simulink model "irep_force_control_m15"  (R2015a)
settings: Solver=ode3  StartTime=0.0  StopTime=inf  FixedStep=dt  RelTol=1e-3
InitFcn:
  | IREP_DEPENDENCY
  | init_omni
  | init_filters
  | init_invivo
  | init_telemanipulation
  | init_parker_xyz
  | init_magnetic_tracker
  | init_loadcell
  | init_scopes
  | init_homing
  | init_force_control
  | init_xpc_invivo_simu
undefined symbols (not defined in the file): ang_vel_scale, B_simu, beta, camera_home_voltage, counter_offset, dt, dt_trakstar, E_Y, encoder_counts, epsilon_robust_inverse, FS_LUT_TAU, FS_LUT_WE, gear_ratio, HomingFineEps, HomingRoughEps, HomingRoughVelocity, I1_primary, I1_secondary, I2_primary, I2_secondary, irep_parameters_left, irep_parameters_right, joystick_filter_coeffs, K_d, K_i, K_naive_inv, K_p, k_right, L1l, L1r, L2l, L2r, L_zeus, left_arm_home_voltage, left_x0_parallelogram, LeftArmHomingDirectionVector, LeftArmHomingIntGain, lin_vel_scale, LOADCELL_BIAS, LOADCELL_GAIN, max_conf_space_speed, N_joystick, N_pots, N_trakstar, OmegaMax, OmegaMin, orientation_epsilon, position_epsilon, pots_filter_coeffs, q_eps_backlash, quadrature_mode, r, right_arm_home_voltage, RightArmHomingDirectionVector, RightArmHomingIntGain, screw_pitch, statics_param, tau_compression_bias, tau_compression_gains, tau_neutral_deadband ... (+16)
libraries: slrtlib x39, simulink x23, xpcobsoletelib x23, xpcconteclib x23, xpcrtudplib x12, xpcmeasurementcomputinglib x6, dspswit3 x2, dspsigops x1
(part 7 of 7)

== matlab function irep_force_control_m15/Trajectory Planner/Right Arm/Low Level/Home Procedure/Fine_Rough_Homing_Switch ==
  data: EnableFineHoming output; error input; dt input; q_des output; ERROR_eps input; HomingVel input; q_cur input; HomedJoint output boolean; PrevHomedJoint input boolean
function [EnableFineHoming,q_des,HomedJoint] = fcn(error, dt,ERROR_eps,HomingVel,q_cur,PrevHomedJoint)
%#eml
%   By Long Wang, 2015/1/20
%   Input:
%       error       -> the current error in potentiometers
%       ERROR_eps   -> the tolenrace defined in potentiometers which will determine if within rough control range 
%       q_cur       -> the previous command
%       PrevHomedJoint  -> if homed detected from the previous time step
%       HomingVel       -> the joint velocity to command if the joint is rough homing mode
HomedJoint = (abs(error)<ERROR_eps);
HomedJoint = (HomedJoint|PrevHomedJoint); 
%   if the joint was detected homed previously, it will be forever seen as homed
%   to avoid noise on pots.
if sum(HomedJoint)==9
    % all joints are in rough homing control range, need to use fine homing
    q_des = q_cur; % stays the previous command
    EnableFineHoming = 1;
else
    %   not all joints are in rough homing control range
    %   the ones which are not, need to give constant velocity command
    %   And the other joints will be waiting untill all the joints are in Fine Homing mode
    EnableFineHoming = 0;
    velocity = (1-HomedJoint).*sign(error).*HomingVel; 
    q_des = q_cur + velocity*dt;
end

== matlab function irep_force_control_m15/Wrench Estimation/Wrench Est Right Arm/compute wrench est ==
  data: Ws output; W_seg1 output; tau_curr input; Psi input; n_t input; n_n input; c_t input; c_n input; L input; r input; statics_param input; probe_offset input
function [Ws,W_seg1] = fcn(tau_curr,Psi,n_t,n_n,c_t,c_n,L,r,statics_param,probe_offset)
%#eml
q = in_vivo_invkin(Psi,r);
[Ws,W_seg1] = ...
    right_arm_wrench_estimation(tau_curr,...
    q,Psi,...
    n_t,n_n,...
    c_t,c_n,...
    L,r,...
    statics_param,...
    probe_offset);

== matlab function irep_force_control_m15/Trajectory Planner/Left Arm/Low Level/Home Procedure/Fine_Rough_Homing_Switch ==
  data: EnableFineHoming output; error input; dt input; q_des output; ERROR_eps input; HomingVel input; q_cur input; HomedJoint output boolean; PrevHomedJoint input boolean
function [EnableFineHoming,q_des,HomedJoint] = fcn(error, dt,ERROR_eps,HomingVel,q_cur,PrevHomedJoint)
%#eml
%   By Long Wang, 2015/1/20
%   Input:
%       error       -> the current error in potentiometers
%       ERROR_eps   -> the tolenrace defined in potentiometers which will determine if within rough control range 
%       q_cur       -> the previous command
%       PrevHomedJoint  -> if homed detected from the previous time step
%       HomingVel       -> the joint velocity to command if the joint is rough homing mode
HomedJoint = (abs(error)<ERROR_eps);
HomedJoint = (HomedJoint|PrevHomedJoint); 
%   if the joint was detected homed previously, it will be forever seen as homed
%   to avoid noise on pots.
if sum(HomedJoint)==9
    % all joints are in rough homing control range, need to use fine homing
    q_des = q_cur; % stays the previous command
    EnableFineHoming = 1;
else
    %   not all joints are in rough homing control range
    %   the ones which are not, need to give constant velocity command
    %   And the other joints will be waiting untill all the joints are in Fine Homing mode
    EnableFineHoming = 0;
    velocity = (1-HomedJoint).*sign(error).*HomingVel; 
    q_des = q_cur + velocity*dt;
end

== matlab function irep_force_control_m15/Trajectory Planner/Left Arm/Low Level/Home Procedure/Homing Flags/Homing Completion ==
  data: u input; Homed output; EPS input; dt input; Homed_T output; Homed_T_prev input
function [Homed,Homed_T] = fcn(u,EPS,dt,Homed_T_prev)
%#eml
Homed_T = zeros(9,1);
u = abs(u);
Homed = (u<=EPS);
for i=1:9
    if Homed(i)
        Homed_T(i) = Homed_T_prev(i) + dt; %increment timer
    else
        Homed_T(i) = 0; % reset timer
    end
end

== matlab function irep_force_control_m15/Trajectory Planner/Left Arm/High Level/Task Space/Desired Twist Module/Compute Twist ==
  data: p_des input; R_des input; MSG_Type input; x_des output; p_curr input; R_curr input; Vmax input; Vmin input; position_epsilon input; lin_vel_scale input; OmegaMax input; OmegaMin input; orientation_epsilon input; ang_vel_scale input; theta output
function [x_des,theta] = fcn(p_des,R_des,MSG_Type,p_curr,R_curr,Vmax,Vmin,position_epsilon,lin_vel_scale,OmegaMax,OmegaMin,orientation_epsilon,ang_vel_scale)
%--------------------------------------------------------------------------
% decode the message_type
% MSG_Type def
% bit0 = valid massage or not(enable or not)
% bit1 = time stamping requested or not (if should send back the local time or not)
enable = bitand(uint8(floor(MSG_Type)),1);
% position
% theta_err = 0;
position_error = p_des-p_curr;
M = norm(position_error);
% orientation
R = R_curr'*R_des;
theta = acos((R(1,1)+R(2,2)+R(3,3)-1)/2);
if isnan(theta)
    theta = 0;
%     theta_err = 1;
end
%----------------------------------------------------------------------
if enable == 1
    if M < position_epsilon && theta < orientation_epsilon
        x_des = zeros(6,1);
    else
        n = position_error/M;
        r_non_unit = [R(3,2)-R(2,3);R(1,3)-R(3,1);R(2,1)-R(1,2)];
        if sum(r_non_unit) == 0
            r = zeros(3,1);
        else
            r = r_non_unit/norm(r_non_unit);
        end
        if M > lin_vel_scale*position_epsilon
            LinVelMag = Vmax; % mm/s
        else
            LinVelMag = M*(Vmax-Vmin)/(position_epsilon*(lin_vel_scale-1)) + (lin_vel_scale*Vmin-Vmax)/(lin_vel_scale-1);
        end
        if theta > ang_vel_scale * orientation_epsilon
            AngVelMag = OmegaMax;
        else
            AngVelMag = theta*(OmegaMax-OmegaMin)/(orientation_epsilon*(ang_vel_scale-1))+ (ang_vel_scale*OmegaMin-OmegaMax)/(ang_vel_scale-1);
        end
        x_des = [LinVelMag*n
                 AngVelMag*r];
    end
else
    x_des = zeros(6,1);
end

== matlab function irep_force_control_m15/Trajectory Planner/Right Arm/High Level/Actuation Compensation/q_eps 5th order poly/Embedded MATLAB Function ==
  data: p_des input; p_curr input; tf input; tc input; p output; pdot output; conf input; confn output; t0 input; t0n output; p0n output; p0 input; enable input
function [p,pdot,confn,t0n,p0n] = fifth_order_p(p_des,p_curr,tf,tc,conf,t0,p0,enable)

if enable == 0                  % Configuration space is not used (pdot = 0). 
    p = p_curr;          % However we do want to record the current 
    confn = 0;                  % position in order to be ready as soon 
    t0n = tc;                   % as the enable becomes 1. 
    p0n = p_curr;
    pdot = zeros(9,1);
else
    if (p_des-p0)'*(p_des-p0) > 0
        if conf == 0                % conf = 0 means that the 5th order poly 
            p0n = p0;               % is not configured for the desired trajectory.
            t0n = tc;               % Therefore, the block is initialized.
            confn = 1;
            p = p0;
            pdot = zeros(9,1);
        else
            p0n = p0;
            t0n = t0;
            confn = conf;
            % 5th order polynomial
            a0 = p0;
            a4 = -15*(p_des-p0);
            a3 = -2/3 * a4;
            a5 = -2/5 * a4;
            t = tc-t0;
            tau = t/tf;
            if t < tf
                p = a0 + a3 * tau^3 + a4 * tau^4 + a5 * tau^5;
                pdot = 3*a3*t^2/tf^3 + 4*a4*t^3/tf^4 + 5*a5*t^4/tf^5;
            else
                p = p_des;
                pdot = zeros(9,1);
                p0n = p_des;
            end
        end
    else
        p = p_des;
        pdot = zeros(9,1);
        confn = 0;
        p0n = p0;
        t0n = t0;
    end
end
%------------------------------------------------------------------------

== matlab function irep_force_control_m15/Trajectory Planner/Right Arm/High Level/Actuation Compensation/RR Act Compensation ==
  data: conf_space input; eps output; q_dot input
function eps= RR_Act_Comp(conf_space,q_dot)
%#codegen
% Edited by Rajarshi Roy
% Last Updated: 12/1/2015
% Compensation initialization
eps = zeros(9,1); 
% Compensation correction
flag_direction = 1; % this flag_direction has been abandoned. not being used.
eps([4,5,6,7],1) = RRComputeActuation(flag_direction,conf_space,q_dot);

== matlab function irep_force_control_m15/Dual daVinci MTM/MTML/Embedded MATLAB Function ==
  data: R_vec input; R output
function R = parse_rot(R_vec)
%#eml
R = reshape(R_vec,3,3);

== matlab function irep_force_control_m15/In-Vivo System/Magnetic Tracker 125 Hz/Process sensors ==
  data: BaseX_sr input; psi output; BaseZ_sr input; Seg1_Z_sr input; Seg2_Z_sr input; theta_eps input; error_flag output
function [psi,error_flag] = fcn(BaseX_sr,BaseZ_sr,Seg1_Z_sr,Seg2_Z_sr,theta_eps)
%#eml
[psi,error_flag] = get_psi_measured_2segments(BaseX_sr,BaseZ_sr,Seg1_Z_sr,Seg2_Z_sr,theta_eps);

== matlab function irep_force_control_m15/Dual daVinci MTM/Task Space Command/Right Arm - 5th Order Polynomial and Slerp/Embedded MATLAB Function1 ==
  data: quat output; quat_f input; quat_curr input; tf input; tc input; conf input; confn output; t0 input; t0n output; quat0n output; quat0 input; enable input; RECORD output
function [quat,confn,t0n,quat0n,RECORD] = quat_slerp(quat_f,quat_curr,tf,tc,conf,t0,quat0,enable)
%%  modified version of 5th order poly for Slerp
%   
RECORD = 0;
if enable == 0                  % Configuration space is not used (pdot = 0). 
    quat = quat_curr;
    confn = 0;                  % position in order to be ready as soon 
    t0n = tc;                   % as the enable becomes 1. 
    quat0n = quat_curr;
else
    if (quat0'*quat_f)<1
        if conf == 0                % conf = 0 means that the 5th order poly 
            quat0n = quat0;               % is not configured for the desired trajectory.
            t0n = tc;               % Therefore, the block is initialized.
            confn = 1;
            quat = quat0;
        else
            quat0n = quat0;
            t0n = t0;
            confn = conf;
            % Slerp
            t = tc-t0;
            tau = t/tf;
            if t < tf
                RECORD = 1;
                quat = slerp(quat0,quat_f,tau);
            else
                quat = quat_f;
                quat0n = quat_f;
            end
        end
    else
        quat = quat_f;
        confn = 0;
        quat0n = quat0;
        t0n = t0;
    end
end
%------------------------------------------------------------------------

== matlab function irep_force_control_m15/Trajectory Planner/Right Arm/High Level/Task Space/pose cur quat ==
  data: R input; quat output
function quat   = convert_rot_to_quat(R)
   quat = rot2quat(R);
end

== matlab function irep_force_control_m15/Dual daVinci MTM/MTMR/Embedded MATLAB Function ==
  data: R_vec input; R output
function R = parse_rot(R_vec)
%#eml
R = reshape(R_vec,3,3);

== matlab function irep_force_control_m15/Dual daVinci MTM/MTMR/Embedded MATLAB Function1 ==
  data: R input; quat output
function quat   = convert_rot_to_quat(R)
   quat = rot2quat(R);
end

== matlab function irep_force_control_m15/Dual daVinci MTM/MTML/Embedded MATLAB Function1 ==
  data: R input; quat output
function quat   = convert_rot_to_quat(R)
   quat = rot2quat(R);
end

== matlab function irep_force_control_m15/Trajectory Planner/Left Arm/High Level/Task Space/pose cur quat ==
  data: R input; quat output
function quat   = convert_rot_to_quat(R)
   quat = rot2quat(R);
end

== matlab function irep_force_control_m15/Trajectory Planner/UDP_SendTo_MTM/Left_UDP/Embedded MATLAB Function ==
  data: R input; R_vec output
function R_vec = R_to_vec(R)
%#eml
%%  This func will cast a [3x3] rotation matrix to [9x1]
%%  The mapping will be column matrix, see for yourself.
R_vec = R(:);

== matlab function irep_force_control_m15/Trajectory Planner/UDP_SendTo_MTM/Left_UDP/MSG_Decoding ==
  data: MSG_Type input; EN output
function EN = Decode(MSG_Type)
%#eml
% decode the message_type
% MSG_Type def
% bit0 = valid massage or not(enable or not)
% bit1 = time stamping requested or not (if should send back the local time or not)
enable = bitand(uint8(floor(MSG_Type)),2);
EN= double(enable);

== matlab function irep_force_control_m15/Trajectory Planner/UDP_SendTo_MTM/Left_UDP/pose convert/Quaternion To Rotation ==
  data: quat input; R output
function R = fcn(quat)
%#eml
if norm(quat)==0
    quat = [1;0;0;0];
end
R = quat2rot(quat);

== matlab function irep_force_control_m15/Trajectory Planner/UDP_SendTo_MTM/Left_UDP/pose_curr_scope/R_to_axis_angle1 ==
  data: R input; n_vec output; theta output
function [n_vec,theta] = AxisAngle(R)
%#eml
% Axis_angle(R) gives the rotation axis and the rotation angle extracted from rotation matrix R
% Note this function handles singular cases even if theta=0 or theta=180
% degrees, which cause the normal axis equation to become undefined.
% Written by N. Simaan
% Last updated 10/14/2012.

cos_theta=(trace(R)-1)/2;
sin_theta=(1/2)*sqrt((R(3,2)-R(2,3))^2 + (R(1,3)-R(3,1))^2 + (R(2,1)-R(1,2))^2);
theta=atan2(sin_theta,cos_theta);
index=0;
if abs(sin_theta)>1e-6 % before it was 1e-12, Long Wang changed it.
    n_cross=1/(2*sin_theta)*(R-R');
    n_vec=[-n_cross(2,3);n_cross(1,3);-n_cross(1,2)]; %disp('aaa');
    n_vec=n_vec/norm(n_vec);
else
    if cos_theta>0  %this means identity matrix
        n_vec=[0;0;0]; %I choose this arbitrarily to designate the special case for identity matrix
    else  %this is the case where theta is 180 degrees
        nx=sqrt((R(1,1)-cos_theta)/(1-cos_theta));
        ny=sqrt((R(2,2)-cos_theta)/(1-cos_theta));
        nz=sqrt((R(3,3)-cos_theta)/(1-cos_theta));
        
        %%% find the axis that best fits the given rotation matrix
        signs=[[1;1;1],...
               [1;-1;1],...
               [1;-1;-1],...
               [1;1;-1],...
               [-1;1;1],...
               [-1;-1;1],...
               [-1;-1;-1],...
               [-1;1;-1]];
        
        e=zeros(1,8); 
        
        for i=1:1:8
            n_candidate=signs(:,i).*[nx;ny;nz];
            Temp=rotd(n_candidate,theta*180/pi), %rotd takes its input in degrees
            e(1,i)=sum(sum((Temp-R).*(Temp-R)));
        end;    
              e,
        e_min=min(e); %the best fit    
        index=0
        for i=1:1:8  %find the index of the combination that produces the closest rotation
            if e(1,i)==e_min 
                index=i;
                break; 
            end;
        end;
        
        n_vec=signs(:,index).*[nx;ny;nz];
    end
end

== matlab function irep_force_control_m15/Wrench Estimation/tau sensing compensation/tau sensing compensation LUT/tau seg2 bias LUT/tau8_bias_neg/MATLAB Function1 ==
  data: theta input; F output; delta input; X input; Y input; V input
function F = fcn(theta,delta,X,Y,V)
%#codegen
F = interp2(X,Y,V,theta,delta);

== matlab function irep_force_control_m15/Wrench Estimation/Wrench Compensation/wrench sensing compensation LUT/wrench seg2 bias LUT/Interp2 Case B/MATLAB Function2 ==
  data: theta input; F output; delta input; X input; Y input; V input
function F = fcn(theta,delta,X,Y,V)
%#codegen
F = interp2(X,Y,V,theta,delta);

== matlab function irep_force_control_m15/Wrench Estimation/Wrench Compensation/wrench sensing compensation LUT/wrench seg2 bias LUT/Interp2 Case B/MATLAB Function4 ==
  data: theta input; F output; delta input; X input; Y input; V input
function F = fcn(theta,delta,X,Y,V)
%#codegen
F = interp2(X,Y,V,theta,delta);

== matlab function irep_force_control_m15/Wrench Estimation/tau sensing compensation/tau sensing compensation LUT/tau seg2 bias LUT/tau8_bias_pos/MATLAB Function2 ==
  data: theta input; F output; delta input; X input; Y input; V input
function F = fcn(theta,delta,X,Y,V)
%#codegen
F = interp2(X,Y,V,theta,delta);

== matlab function irep_force_control_m15/Wrench Estimation/tau sensing compensation/tau sensing compensation LUT/tau seg2 bias LUT/tau7_bias_pos/MATLAB Function2 ==
  data: theta input; F output; delta input; X input; Y input; V input
function F = fcn(theta,delta,X,Y,V)
%#codegen
F = interp2(X,Y,V,theta,delta);

== matlab function irep_force_control_m15/Wrench Estimation/tau sensing compensation/tau sensing compensation LUT/tau seg2 bias LUT/tau7_bias_neg/MATLAB Function1 ==
  data: theta input; F output; delta input; X input; Y input; V input
function F = fcn(theta,delta,X,Y,V)
%#codegen
F = interp2(X,Y,V,theta,delta);

== matlab function irep_force_control_m15/Wrench Estimation/tau sensing compensation/tau sensing compensation LUT/tau seg2 bias LUT/tau6_bias_pos/MATLAB Function2 ==
  data: theta input; F output; delta input; X input; Y input; V input
function F = fcn(theta,delta,X,Y,V)
%#codegen
F = interp2(X,Y,V,theta,delta);

== matlab function irep_force_control_m15/Wrench Estimation/tau sensing compensation/tau sensing compensation LUT/tau seg2 bias LUT/tau6_bias_neg/MATLAB Function1 ==
  data: theta input; F output; delta input; X input; Y input; V input
function F = fcn(theta,delta,X,Y,V)
%#codegen
F = interp2(X,Y,V,theta,delta);

== matlab function irep_force_control_m15/Wrench Estimation/tau sensing compensation/tau sensing compensation LUT/tau seg2 bias LUT/tau5_bias_pos/MATLAB Function2 ==
  data: theta input; F output; delta input; X input; Y input; V input
function F = fcn(theta,delta,X,Y,V)
%#codegen
F = interp2(X,Y,V,theta,delta);

== matlab function irep_force_control_m15/Wrench Estimation/tau sensing compensation/tau sensing compensation LUT/tau seg2 bias LUT/tau5_bias_neg/MATLAB Function1 ==
  data: theta input; F output; delta input; X input; Y input; V input
function F = fcn(theta,delta,X,Y,V)
%#codegen
F = interp2(X,Y,V,theta,delta);

== matlab function irep_force_control_m15/Wrench Estimation/Wrench Compensation/wrench sensing compensation LUT/wrench seg2 bias LUT/Interp2 Case A/MATLAB Function1 ==
  data: theta input; F output; delta input; X input; Y input; V input
function F = fcn(theta,delta,X,Y,V)
%#codegen
F = interp2(X,Y,V,theta,delta);

== matlab function irep_force_control_m15/Wrench Estimation/Wrench Compensation/wrench sensing compensation LUT/wrench seg2 bias LUT/Interp2 Case A/MATLAB Function2 ==
  data: theta input; F output; delta input; X input; Y input; V input
function F = fcn(theta,delta,X,Y,V)
%#codegen
F = interp2(X,Y,V,theta,delta);

== matlab function irep_force_control_m15/Wrench Estimation/Wrench Compensation/wrench sensing compensation LUT/wrench seg2 bias LUT/Interp2 Case A/MATLAB Function4 ==
  data: theta input; F output; delta input; X input; Y input; V input
function F = fcn(theta,delta,X,Y,V)
%#codegen
F = interp2(X,Y,V,theta,delta);

== matlab function irep_force_control_m15/Wrench Estimation/Wrench Compensation/wrench sensing compensation LUT/wrench seg2 bias LUT/Interp2 Case C/MATLAB Function1 ==
  data: theta input; F output; delta input; X input; Y input; V input
function F = fcn(theta,delta,X,Y,V)
%#codegen
F = interp2(X,Y,V,theta,delta);

== matlab function irep_force_control_m15/Wrench Estimation/Wrench Compensation/wrench sensing compensation LUT/wrench seg2 bias LUT/Interp2 Case C/MATLAB Function2 ==
  data: theta input; F output; delta input; X input; Y input; V input
function F = fcn(theta,delta,X,Y,V)
%#codegen
F = interp2(X,Y,V,theta,delta);

== matlab function irep_force_control_m15/Wrench Estimation/Wrench Compensation/wrench sensing compensation LUT/wrench seg2 bias LUT/Interp2 Case C/MATLAB Function4 ==
  data: theta input; F output; delta input; X input; Y input; V input
function F = fcn(theta,delta,X,Y,V)
%#codegen
F = interp2(X,Y,V,theta,delta);

== matlab function irep_force_control_m15/Wrench Estimation/Wrench Compensation/wrench sensing compensation LUT/wrench seg2 bias LUT/Interp2 Case D/MATLAB Function1 ==
  data: theta input; F output; delta input; X input; Y input; V input
function F = fcn(theta,delta,X,Y,V)
%#codegen
F = interp2(X,Y,V,theta,delta);

== matlab function irep_force_control_m15/Wrench Estimation/Wrench Compensation/wrench sensing compensation LUT/wrench seg2 bias LUT/Interp2 Case D/MATLAB Function2 ==
  data: theta input; F output; delta input; X input; Y input; V input
function F = fcn(theta,delta,X,Y,V)
%#codegen
F = interp2(X,Y,V,theta,delta);

== matlab function irep_force_control_m15/Wrench Estimation/Wrench Compensation/wrench sensing compensation LUT/wrench seg2 bias LUT/Interp2 Case D/MATLAB Function4 ==
  data: theta input; F output; delta input; X input; Y input; V input
function F = fcn(theta,delta,X,Y,V)
%#codegen
F = interp2(X,Y,V,theta,delta);
